simulink model "linear_model"
settings: Solver=ode45  StartTime=0.0  StopTime=20  RelTol=1e-3
values from neighbouring files (symbols this model uses):
  Alin = eval(Alin)    [main.m]    (also in matlab.mat = [0 0 0 0 0 0 14.3782406735 -97.1270102365 1 0 -8.0820897902 ; stav_lin.mat = [0 0 0 0 0 0 5.28235362921 -73.758221558 1 0 -6.9230827764 9; stavova_zpetna.m; workspace.mat = [0 0 0 0 0 0 5.28235362921 -73.758221558 1 0 -6.9230827764 9)
  Blin = eval(Blin)    [main.m]    (also in matlab.mat = [0 0 32.1730635168 -49.2662800726]; stav_lin.mat = [0 0 13.3327451106 -18.0997049117]; stavova_zpetna.m; workspace.mat = [0 0 13.3327451106 -18.0997049117])
  Clin = subs(Clin, xs, xps)    [main.m]    (also in matlab.mat = [1  0  0  0; 0  1  0  0]; stavova_zpetna.m = eval(Clin); workspace.mat = [1  0  0  0; 0  1  0  0])
  Dlin = subs(Dlin, us, ups)    [main.m]    (also in matlab.mat = [0 0]; stavova_zpetna.m = eval(Dlin); workspace.mat = [0 0])
settings Model: Creator=Matous  LastModifiedBy=matous
settings DataIOCC: LimitDataPoints=on  SaveFormat=Array  ReturnWorkspaceOutputs=off
settings OptimizationCC: LifeSpan=inf  SimCompilerOptimization=Off
settings DebuggingCC: SolverPrmCheckMsg=warning  MultiTaskDSMMsg=warning  MultiTaskCondExecSysMsg=none  FcnCallInpInsideContextMsg=Enable All  FrameProcessingCompatibilityMsg=warning  StrictBusMsg=None  SFUnexpectedBacktrackingDiag=warning  SFNoUnconditionalDefaultTransitionDiag=warning
settings HardwareCC: ProdBitPerPointer=32  ProdLargestAtomicFloat=None  ProdIntDivRoundTo=Undefined  ProdEndianess=Unspecified  ProdWordSize=32  ProdHWDeviceType=32-bit Generic
settings ModelReferenceCC: PropagateSignalLabelsOutOfModel=off
settings SFSimCC: SimUseLocalCustomCode=off
settings RTWCC: RTWUseLocalCustomCode=off  IncludeERTFirstTime=on  RTWCompilerOptimization=Off
settings GRTTargetCC: GeneratePreprocessorConditionals=Disable all

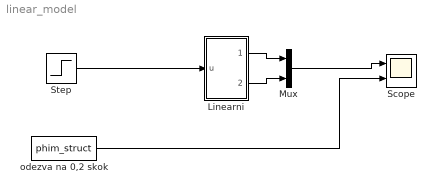
== system linear_model ==
  Linearni : Subsystem
  Mux : Mux  Inputs=2
  Scope : Scope  NumInputPorts=2
      settings: YMin=-5~-5  YMax=5~5
  Step : Step  After=-0.02  SampleTime=0
  odezva na 0,2 skok : FromWorkspace  VariableName=phim_struct  SampleTime=0
  wires:
  Step/1 -> Linearni/1(u)
  Mux/1 -> Scope/1
  Linearni/1(phim) -> Mux/1
  Linearni/2(phip) -> Mux/2
  odezva na 0,2 skok/1 -> Scope/2

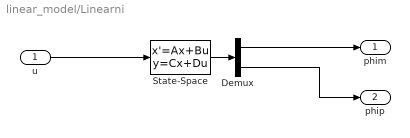
== system linear_model/Linearni ==
  u : Inport
  Demux : Demux  Outputs=2
  State-Space : StateSpace  A=Alin  B=Blin  C=Clin  D=Dlin
  phim : Outport
  phip : Outport  Port=2
  wires:
  Demux/1 -> phim/1
  u/1 -> State-Space/1
  State-Space/1 -> Demux/1
  Demux/2 -> phip/1
